simulink model "Simulink_Klostermair4"  (R2024a)
settings: Solver=ode4  StartTime=0.0  StopTime=3  FixedStep=0.001  RelTol=1e-05  AbsTol=1e-08
values from neighbouring files (symbols this model uses):
  g = 9.81    [Assignment4_2.m]    (also in ssignment4_additional.m)
  h = 0.2    [Assignment4_2.m]    (also in ssignment4_additional.m)
  k_max = 150    [ssignment4_additional.m]
  k_min = 50    [ssignment4_additional.m]
  x_max = -0.6*l0    (= -0.6)    [ssignment4_additional.m]
undefined symbols (not defined in the file or in its folder): magnitude
libraries: simulink x1
settings Model: Creator=Luki_2000  LastModifiedBy=Luki_2000

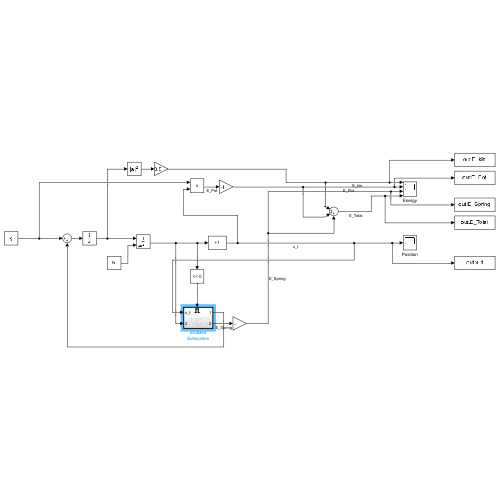
[thumbnail: Simulink's stored preview of the top-level diagram]
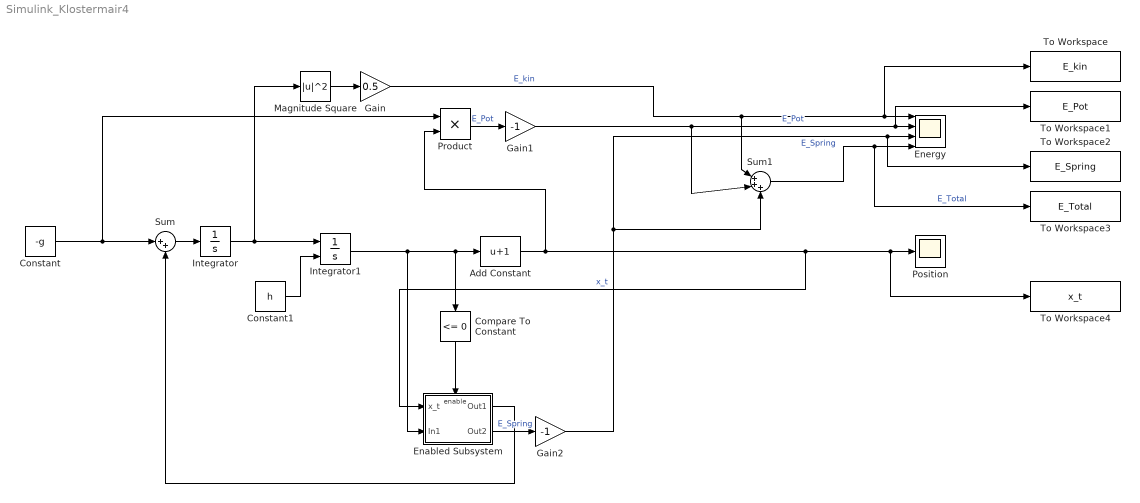
== system Simulink_Klostermair4 ==
  Add Constant : Bias  Bias=1  SaturateOnIntegerOverflow=off
  Compare To Constant : simulink/Logic and Bit Operations/Compare To Constant  relop=<=  const=0  OutDataTypeStr=boolean
  Constant : Constant  Value=-g
  Constant1 : Constant  Value=h
  Enabled Subsystem : Subsystem  TreatAsAtomicUnit=on
  Energy : Scope  NumInputPorts=4
  Gain : Gain  Gain=0.5
  Gain1 : Gain  Gain=-1
  Gain2 : Gain  Gain=-1
  Integrator : Integrator
  Integrator1 : Integrator  InitialConditionSource=external
  Magnitude Square : Math  Operator=magnitude^2  SignedPower=on  RndMeth=Zero
  Position : Scope
  Product : Product
  Sum : Sum  Inputs=|++
  Sum1 : Sum  Inputs=|+++
  To Workspace : ToWorkspace  VariableName=E_kin  SaveFormat=Timeseries  SampleTime=-1
  To Workspace1 : ToWorkspace  VariableName=E_Pot  SaveFormat=Timeseries  SampleTime=-1
  To Workspace2 : ToWorkspace  VariableName=E_Spring  SaveFormat=Timeseries  SampleTime=-1
  To Workspace3 : ToWorkspace  VariableName=E_Total  SaveFormat=Timeseries  SampleTime=-1
  To Workspace4 : ToWorkspace  VariableName=x_t  SaveFormat=Timeseries  SampleTime=-1
  wires:
  Constant/1 -> Product/1, Sum/1
  Sum/1 -> Integrator/1
  Constant1/1 -> Integrator1/2
  Integrator/1 -> Magnitude Square/1, Integrator1/1
  Integrator1/1 -> Enabled Subsystem/2(In1), Compare To Constant/1, Add Constant/1
  Compare To Constant/1 -> Enabled Subsystem/Enable
  Magnitude Square/1 -> Gain/1
  Add Constant/1 -> Product/2, Enabled Subsystem/1(x_t), To Workspace4/1, Position/1  "x_t"
  Enabled Subsystem/1(Out1) -> Sum/2
  Gain/1 -> Sum1/1, To Workspace/1, Energy/1  "E_kin"
  Sum1/1 -> To Workspace3/1, Energy/4  "E_Total"
  Product/1 -> Gain1/1  "E_Pot"
  Gain1/1 -> Sum1/2, To Workspace1/1, Energy/2  "E_Pot"
  Enabled Subsystem/2(Out2) -> Gain2/1  "E_Spring"
  Gain2/1 -> Sum1/3, To Workspace2/1, Energy/3  "E_Spring"

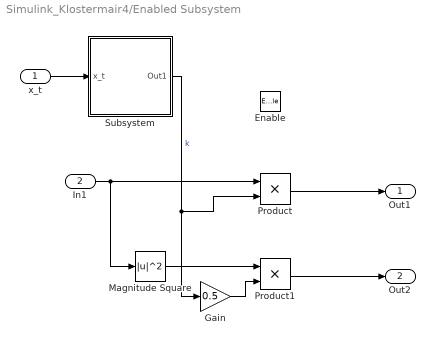
== system Simulink_Klostermair4/Enabled Subsystem ==
  x_t : Inport
  In1 : Inport  Port=2
  Enable : EnablePort
  Gain : Gain  Gain=0.5
  Magnitude Square : Math  Operator=magnitude^2  SignedPower=on  RndMeth=Zero
  Product : Product
  Product1 : Product
  Subsystem : Subsystem
  Out1 : Outport
  Out2 : Outport  Port=2
  wires:
  In1/1 -> Magnitude Square/1, Product/1
  Subsystem/1(Out1) -> Gain/1, Product/2  "k"
  Product/1 -> Out1/1
  Product1/1 -> Out2/1
  Magnitude Square/1 -> Product1/1
  Gain/1 -> Product1/2
  x_t/1 -> Subsystem/1(x_t)

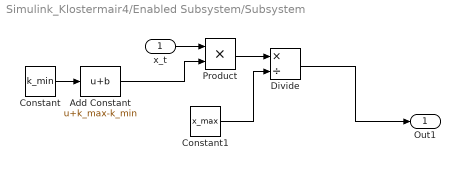
== system Simulink_Klostermair4/Enabled Subsystem/Subsystem ==
  x_t : Inport
  Add Constant : Bias  Bias=k_max-k_min  SaturateOnIntegerOverflow=off
  Constant : Constant  Value=k_min
  Constant1 : Constant  Value=x_max
  Divide : Product  Inputs=*/
  Product : Product
  Out1 : Outport
  wires:
  x_t/1 -> Product/1
  Constant/1 -> Add Constant/1
  Add Constant/1 -> Product/2
  Product/1 -> Divide/1
  Constant1/1 -> Divide/2
  Divide/1 -> Out1/1
